simulink model "sampleModel1415"  (R2023a)
settings: Solver=VariableStepAuto  StartTime=0.0  StopTime=10.0  RelTol=1e-3
libraries: hdlsllib x7, simulink x4
settings Model: Creator=user1  LastModifiedBy=user1

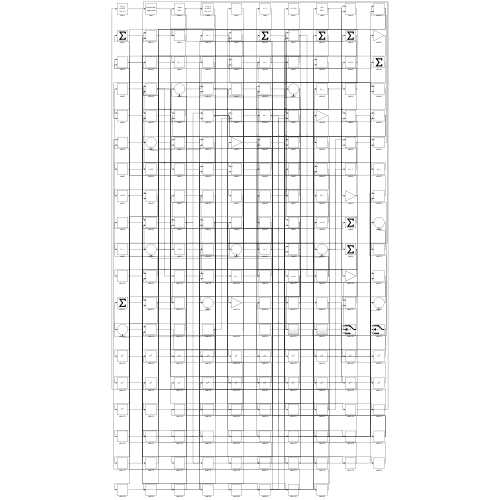
[thumbnail: Simulink's stored preview of the top-level diagram]
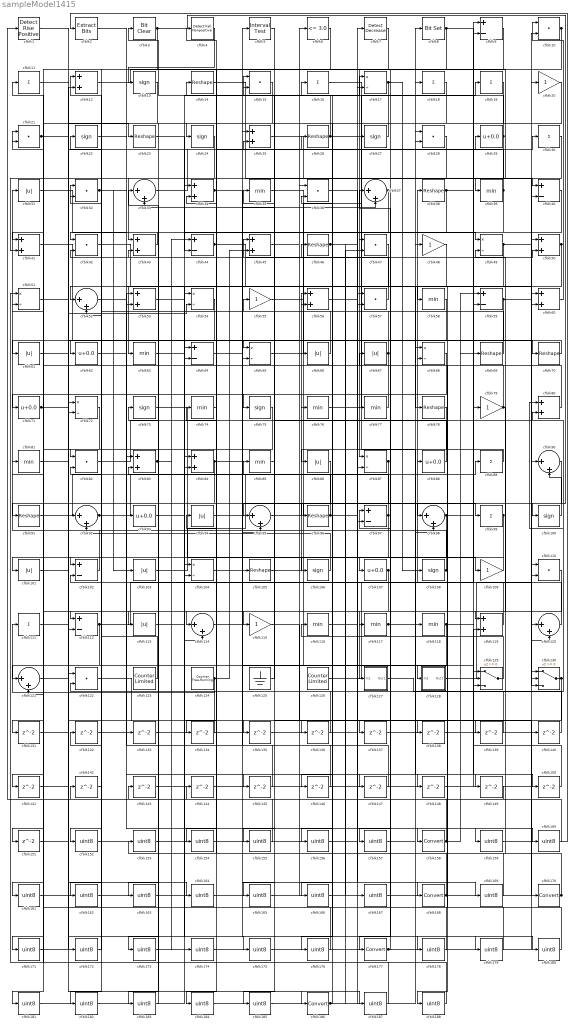
== system sampleModel1415 ==
  cfblk1 : hdlsllib/Logic and Bit Operations/Detect Rise Positive  vinit=0  OutDataTypeStr=boolean
  cfblk{10,15,21,28,32,36,42,47,57,82,110,122} (12 alike) : DotProduct  OutDataTypeStr=Inherit: Inherit via internal rule
  cfblk{13,22,24,27,73,75,100,106,108} (9 alike) : Signum
  cfblk{31,61,66..67,86,94,101,103,113} (9 alike) : Abs  SaturateOnIntegerOverflow=off
  cfblk{9,40,44,59,64,97,102,112} (8 alike) : Sum  Inputs=+-
  cfblk{17,49,51,54,65,68,72,87,104} (9 alike) : Product  Inputs=*/  RndMeth=Zero  SaturateOnIntegerOverflow=on
  cfblk{14,23,26,38,46,69..70,78,91,96,105} (11 alike) : Reshape
  cfblk{29,62,71,88,93,107} (6 alike) : Bias  Bias=0.0  SaturateOnIntegerOverflow=off
  cfblk{20,48,55,79,109,115} (6 alike) : Gain
  cfblk{11,16,18..19,30,89,99,111} (8 alike) : Sum  Inputs=+
  cfblk{33,37,52,90,92,95,98,114,120..121} (10 alike) : Sum  Inputs=|++
  cfblk{35,39,58,63,74,76..77,81,85,116..118} (12 alike) : MinMax
  cfblk{12,25,34,41,43,45,50,53,56,60,80,83..84,119} (14 alike) : Sum
  cfblk123 : hdlsllib/Sources/Counter Limited  uplimit=7  tsamp=-1
  cfblk124 : hdlsllib/Sources/Counter Free-Running  NumBits=16  tsamp=-1
  cfblk125 : Ground
  cfblk126 : hdlsllib/Sources/Counter Limited  uplimit=7  tsamp=-1
  cfblk127 : Subsystem
      settings: LibrarySourceBlock=|
      | hdlsllib/Ports &
      | Subsystems/Subsystem
  cfblk128 : Subsystem
      settings: LibrarySourceBlock=|
      | hdlsllib/Ports &
      | Subsystems/Subsystem
  cfblk129 : Switch  SaturateOnIntegerOverflow=off  InputSameDT=off
  cfblk130 : Switch  SaturateOnIntegerOverflow=off  InputSameDT=off
  cfblk{131..151} (21 alike) : Delay  SampleTime=1
  cfblk{152..157,159..167,169,171..176,178..185,187..188} (32 alike) : DataTypeConversion  OutDataTypeStr=uint8  SaturateOnIntegerOverflow=off  RndMeth=Floor
  cfblk{158,168,170,177,186} (5 alike) : DataTypeConversion  SaturateOnIntegerOverflow=off  RndMeth=Floor
  cfblk2 : simulink/Logic and Bit Operations/Extract Bits  bitsToExtract=Upper half  numBits=8  bitIdxRange=[0 7]  outScalingMode=Preserve fixed-point scaling
      settings: LibrarySourceBlock=|
      | hdlsllib/Logic and Bit
      | Operations/Extract Bits
  cfblk3 : simulink/Logic and Bit Operations/Bit Clear  iBit=0
      settings: LibrarySourceBlock=|
      | hdlsllib/Logic and Bit
      | Operations/Bit Clear
  cfblk4 : hdlsllib/Logic and Bit Operations/Detect Fall Nonpositive  vinit=0  OutDataTypeStr=boolean
  cfblk5 : hdlsllib/Logic and Bit Operations/Interval Test  IntervalClosedRight=on  uplimit=0.5  IntervalClosedLeft=on  lowlimit=-0.5  OutDataTypeStr=boolean
  cfblk6 : hdlsllib/Logic and Bit Operations/Compare To Constant  relop=<=  const=3.0  OutDataTypeStr=boolean
  cfblk7 : simulink/Logic and Bit Operations/Detect Decrease  vinit=0.0  OutDataTypeStr=boolean
      settings: LibrarySourceBlock=|
      | hdlsllib/Logic and Bit
      | Operations/Detect
      | Decrease
  cfblk8 : simulink/Logic and Bit Operations/Bit Set  iBit=0
      settings: LibrarySourceBlock=|
      | hdlsllib/Logic and Bit
      | Operations/Bit Set
  wires:
  cfblk55/1 -> cfblk107/1
  cfblk76/1 -> cfblk19/1
  cfblk12/1 -> cfblk39/1
  cfblk50/1 -> cfblk63/1, cfblk52/1
  cfblk126/1 -> cfblk38/1
  cfblk102/1 -> cfblk31/1
  cfblk26/1 -> cfblk15/1, cfblk130/3
  cfblk60/1 -> cfblk10/1
  cfblk3/1 -> cfblk100/1, cfblk52/2
  cfblk32/1 -> cfblk103/1, cfblk59/2, cfblk135/1
  cfblk73/1 -> cfblk109/1
  cfblk35/1 -> cfblk128/1(In1)
  cfblk91/1 -> cfblk85/1
  cfblk127/1(Out1) -> cfblk80/1
  cfblk109/1 -> cfblk102/1
  cfblk47/1 -> cfblk115/1
  cfblk119/1 -> cfblk73/1
  cfblk58/1 -> cfblk61/1
  cfblk130/1 -> cfblk80/2, cfblk185/1
  cfblk27/1 -> cfblk24/1
  cfblk97/1 -> cfblk35/1, cfblk112/2
  cfblk87/1 -> cfblk83/2, cfblk181/1
  cfblk83/1 -> cfblk44/1, cfblk174/1
  cfblk99/1 -> cfblk131/1, cfblk176/1
  cfblk92/1 -> cfblk88/1, cfblk145/1
  cfblk68/1 -> cfblk177/1
  cfblk128/1(Out1) -> cfblk50/1
  cfblk65/1 -> cfblk29/1
  cfblk15/1 -> cfblk112/1
  cfblk22/1 -> cfblk53/2
  cfblk94/1 -> cfblk56/1
  cfblk19/1 -> cfblk71/1
  cfblk37/1 -> cfblk44/2, cfblk184/1
  cfblk43/1 -> cfblk42/1
  cfblk95/1 -> cfblk99/1
  cfblk98/1 -> cfblk9/1, cfblk117/1, cfblk59/1
  cfblk11/1 -> cfblk72/1
  cfblk23/1 -> cfblk49/1
  cfblk17/1 -> cfblk87/1, cfblk108/1
  cfblk84/1 -> cfblk105/1, cfblk96/1, cfblk91/1
  cfblk122/1 -> cfblk170/1
  cfblk4/1 -> cfblk13/1
  cfblk21/1 -> cfblk23/1, cfblk136/1
  cfblk16/1 -> cfblk118/1
  cfblk25/1 -> cfblk79/1
  cfblk107/1 -> cfblk127/1(In1), cfblk161/1
  cfblk82/1 -> cfblk60/1
  cfblk120/1 -> cfblk12/1
  cfblk33/1 -> cfblk5/1
  cfblk14/1 -> cfblk40/1
  cfblk124/1 -> cfblk111/1, cfblk45/2
  cfblk125/1 -> cfblk45/1
  cfblk118/1 -> cfblk150/1, cfblk151/1
  cfblk69/1 -> cfblk32/1
  cfblk103/1 -> cfblk89/1
  cfblk108/1 -> cfblk11/1, cfblk33/2
  cfblk100/1 -> cfblk90/2
  cfblk9/1 -> cfblk41/1
  cfblk114/1 -> cfblk129/2
  cfblk31/1 -> cfblk93/1
  cfblk79/1 -> cfblk119/1, cfblk21/2
  cfblk70/1 -> cfblk62/1
  cfblk44/1 -> cfblk50/2, cfblk130/2, cfblk78/1, cfblk98/2
  cfblk112/1 -> cfblk9/2, cfblk121/1
  cfblk88/1 -> cfblk15/2
  cfblk105/1 -> cfblk76/1
  cfblk8/1 -> cfblk40/2, cfblk162/1
  cfblk116/1 -> cfblk168/1
  cfblk71/1 -> cfblk30/1, cfblk101/1
  cfblk53/1 -> cfblk34/1
  cfblk39/1 -> cfblk95/1, cfblk4/1
  cfblk10/1 -> cfblk47/1, cfblk157/1
  cfblk34/1 -> cfblk37/2, cfblk58/1, cfblk169/1
  cfblk24/1 -> cfblk41/2
  cfblk90/1 -> cfblk113/1
  cfblk49/1 -> cfblk60/2, cfblk188/1
  cfblk38/1 -> cfblk129/3, cfblk57/2, cfblk82/1
  cfblk41/1 -> cfblk70/1
  cfblk51/1 -> cfblk186/1
  cfblk30/1 -> cfblk106/1
  cfblk29/1 -> cfblk3/1, cfblk43/1
  cfblk77/1 -> cfblk75/1
  cfblk111/1 -> cfblk54/2
  cfblk106/1 -> cfblk92/2
  cfblk6/1 -> cfblk114/1
  cfblk40/1 -> cfblk77/1
  cfblk129/1 -> cfblk16/1
  cfblk117/1 -> cfblk97/1, cfblk149/1
  cfblk46/1 -> cfblk139/1, cfblk167/1
  cfblk2/1 -> cfblk158/1
  cfblk57/1 -> cfblk22/1
  cfblk67/1 -> cfblk26/1, cfblk33/1, cfblk121/2
  cfblk78/1 -> cfblk97/2
  cfblk123/1 -> cfblk42/2
  cfblk59/1 -> cfblk130/1, cfblk182/1
  cfblk89/1 -> cfblk86/1
  cfblk93/1 -> cfblk17/1
  cfblk1/1 -> cfblk65/1
  cfblk13/1 -> cfblk72/2
  cfblk96/1 -> cfblk55/1, cfblk98/1, cfblk146/1
  cfblk66/1 -> cfblk25/2
  cfblk80/1 -> cfblk21/1
  cfblk42/1 -> cfblk114/2
  cfblk45/1 -> cfblk6/1
  cfblk54/1 -> cfblk84/2
  cfblk132/1 -> cfblk65/2
  cfblk62/1 -> cfblk133/1
  cfblk133/1 -> cfblk95/2
  cfblk86/1 -> cfblk134/1
  cfblk134/1 -> cfblk53/1
  cfblk135/1 -> cfblk87/2
  cfblk136/1 -> cfblk84/1
  cfblk115/1 -> cfblk137/1
  cfblk137/1 -> cfblk120/1
  cfblk56/1 -> cfblk138/1
  cfblk138/1 -> cfblk10/2
  cfblk139/1 -> cfblk102/2
  cfblk140/1 -> cfblk36/2
  cfblk75/1 -> cfblk141/1
  cfblk141/1 -> cfblk92/1
  cfblk142/1 -> cfblk32/2
  cfblk143/1 -> cfblk90/1
  cfblk144/1 -> cfblk17/2
  cfblk145/1 -> cfblk83/1
  cfblk146/1 -> cfblk34/2
  cfblk63/1 -> cfblk147/1
  cfblk147/1 -> cfblk25/1
  cfblk52/1 -> cfblk148/1
  cfblk148/1 -> cfblk119/2
  cfblk149/1 -> cfblk1/1
  cfblk150/1 -> cfblk129/1
  cfblk151/1 -> cfblk12/2
  cfblk7/1 -> cfblk152/1
  cfblk152/1 -> cfblk66/1
  cfblk153/1 -> cfblk7/1
  cfblk74/1 -> cfblk154/1
  cfblk154/1 -> cfblk94/1
  cfblk5/1 -> cfblk155/1
  cfblk155/1 -> cfblk74/1
  cfblk48/1 -> cfblk156/1
  cfblk156/1 -> cfblk56/2
  cfblk157/1 -> cfblk48/1
  cfblk158/1 -> cfblk144/1, cfblk82/2, cfblk69/1
  cfblk36/1 -> cfblk159/1
  cfblk159/1 -> cfblk2/1
  cfblk104/1 -> cfblk160/1
  cfblk160/1 -> cfblk142/1
  cfblk161/1 -> cfblk104/1
  cfblk162/1 -> cfblk104/2
  cfblk110/1 -> cfblk163/1
  cfblk163/1 -> cfblk36/1
  cfblk121/1 -> cfblk164/1
  cfblk164/1 -> cfblk110/1
  cfblk85/1 -> cfblk165/1
  cfblk165/1 -> cfblk110/2
  cfblk20/1 -> cfblk166/1
  cfblk166/1 -> cfblk140/1
  cfblk167/1 -> cfblk20/1
  cfblk168/1 -> cfblk153/1, cfblk43/2
  cfblk169/1 -> cfblk116/1
  cfblk170/1 -> cfblk37/1, cfblk49/2, cfblk14/1
  cfblk72/1 -> cfblk171/1
  cfblk171/1 -> cfblk122/1
  cfblk61/1 -> cfblk172/1
  cfblk172/1 -> cfblk122/2
  cfblk18/1 -> cfblk173/1
  cfblk173/1 -> cfblk54/1
  cfblk174/1 -> cfblk18/1
  cfblk81/1 -> cfblk175/1
  cfblk175/1 -> cfblk57/1
  cfblk176/1 -> cfblk81/1
  cfblk177/1 -> cfblk67/1, cfblk120/2
  cfblk131/1 -> cfblk178/1
  cfblk178/1 -> cfblk68/1
  cfblk113/1 -> cfblk179/1
  cfblk179/1 -> cfblk68/2
  cfblk64/1 -> cfblk180/1
  cfblk180/1 -> cfblk132/1
  cfblk181/1 -> cfblk64/1
  cfblk182/1 -> cfblk64/2
  cfblk28/1 -> cfblk183/1
  cfblk183/1 -> cfblk143/1
  cfblk184/1 -> cfblk28/1
  cfblk185/1 -> cfblk28/2
  cfblk186/1 -> cfblk27/1, cfblk47/2, cfblk8/1, cfblk46/1
  cfblk101/1 -> cfblk187/1
  cfblk187/1 -> cfblk51/1
  cfblk188/1 -> cfblk51/2

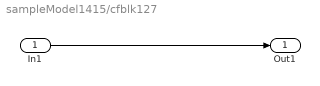
== system sampleModel1415/cfblk127 ==
  In1 : Inport
  Out1 : Outport
  wires:
  In1/1 -> Out1/1

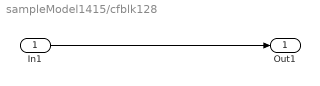
== system sampleModel1415/cfblk128 ==
  In1 : Inport
  Out1 : Outport
  wires:
  In1/1 -> Out1/1
